simulink model "SIMULINK"  (R2023a)
settings: Solver=VariableStepAuto  StartTime=0.0  StopTime=STOP  MaxStep=0.1  MinStep=0.01  RelTol=1e-3
values from neighbouring files (symbols this model uses):
  a = pars(1,1)    [simulinkmodel.m]
  a1 = 0.02    [Izhikevich.m]    (also in simulinkmodel.m = pars(2,1))
  a2 = 0.1    [Izhikevich.m]    (also in simulinkmodel.m = pars(3,1))
  b = normalize(V_feedback)    [interconnection.m]    (also in simulinkmodel.m = pars(1,2))
  b1 = 0.2    [Izhikevich.m]    (also in simulinkmodel.m = pars(2,2))
  b2 = 0.2    [Izhikevich.m]    (also in simulinkmodel.m = pars(3,2))
  c = pars(1,3)    [simulinkmodel.m]
  c1 = -65    [Izhikevich.m]    (also in simulinkmodel.m = pars(2,3))
  c2 = -65    [Izhikevich.m]    (also in simulinkmodel.m = pars(3,3))
  d = pars(1,4)    [simulinkmodel.m]
  d1 = 8    [Izhikevich.m]    (also in simulinkmodel.m = pars(2,4))
  d2 = 2    [Izhikevich.m]    (also in simulinkmodel.m = pars(3,4))
  STOP = 500    [simulinkmodel.m]
settings Model: Creator=HP  LastModifiedBy=HP
settings SolverCC: InitialStep=Auto

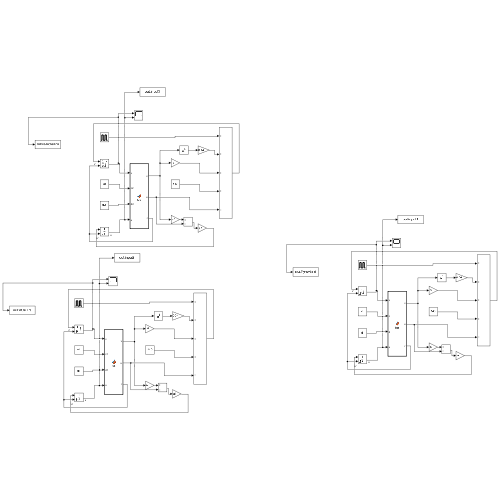
[thumbnail: Simulink's stored preview of the top-level diagram]
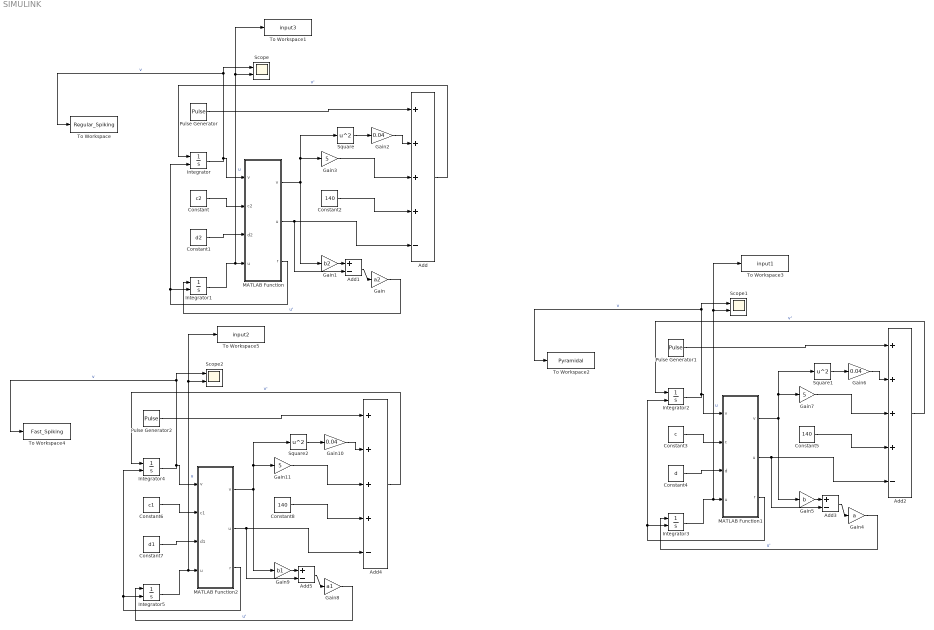
== system SIMULINK ==
  Add : Sum  Inputs=++++-
  Add1 : Sum  Inputs=+-
  Add2 : Sum  Inputs=++++-
  Add3 : Sum  Inputs=+-
  Add4 : Sum  Inputs=++++-
  Add5 : Sum  Inputs=+-
  Constant : Constant  Value=c2
  Constant1 : Constant  Value=d2
  Constant2 : Constant  Value=140
  Constant3 : Constant  Value=c
  Constant4 : Constant  Value=d
  Constant5 : Constant  Value=140
  Constant6 : Constant  Value=c1
  Constant7 : Constant  Value=d1
  Constant8 : Constant  Value=140
  Gain : Gain  Gain=a2
  Gain1 : Gain  Gain=b2
  Gain10 : Gain  Gain=0.04
  Gain11 : Gain  Gain=5
  Gain2 : Gain  Gain=0.04
  Gain3 : Gain  Gain=5
  Gain4 : Gain  Gain=a
  Gain5 : Gain  Gain=b
  Gain6 : Gain  Gain=0.04
  Gain7 : Gain  Gain=5
  Gain8 : Gain  Gain=a1
  Gain9 : Gain  Gain=b1
  Integrator : Integrator  ExternalReset=rising  InitialCondition=c  LimitOutput=on  UpperSaturationLimit=30
  Integrator1 : Integrator  ExternalReset=rising  InitialCondition=d
  Integrator2 : Integrator  ExternalReset=rising  InitialCondition=c  LimitOutput=on  UpperSaturationLimit=30
  Integrator3 : Integrator  ExternalReset=rising  InitialCondition=d
  Integrator4 : Integrator  ExternalReset=rising  InitialCondition=c  LimitOutput=on  UpperSaturationLimit=30
  Integrator5 : Integrator  ExternalReset=rising  InitialCondition=d
  MATLAB Function : MATLAB Function  TreatAsAtomicUnit=on
  MATLAB Function1 : MATLAB Function  TreatAsAtomicUnit=on
  MATLAB Function2 : MATLAB Function  TreatAsAtomicUnit=on
  Pulse Generator : DiscretePulseGenerator  PulseType=Time based  Amplitude=20  Period=STOP/2  PulseWidth=50  PhaseDelay=40
  Pulse Generator1 : DiscretePulseGenerator  PulseType=Time based  Amplitude=20  Period=STOP/2  PulseWidth=50  PhaseDelay=40
  Pulse Generator2 : DiscretePulseGenerator  PulseType=Time based  Amplitude=20  Period=STOP/2  PulseWidth=50  PhaseDelay=40
  Scope : Scope  NumInputPorts=2
  Scope1 : Scope  NumInputPorts=2
  Scope2 : Scope  NumInputPorts=2
  Square : Math  Operator=square
  Square1 : Math  Operator=square
  Square2 : Math  Operator=square
  To Workspace : ToWorkspace  VariableName=Regular_Spiking  SampleTime=-1
  To Workspace1 : ToWorkspace  VariableName=input3  SampleTime=-1
  To Workspace2 : ToWorkspace  VariableName=Pyramidal  SampleTime=-1
  To Workspace3 : ToWorkspace  VariableName=input1  SampleTime=-1
  To Workspace4 : ToWorkspace  VariableName=Fast_Spiking  SampleTime=-1
  To Workspace5 : ToWorkspace  VariableName=input2  SampleTime=-1
  wires:
  Integrator/1 -> To Workspace/1, Scope/1, MATLAB Function/1("v ")  "v"
  Add/1 -> Integrator/1  "v'"
  Gain/1 -> Integrator1/1  "u'"
  Square/1 -> Gain2/1
  Pulse Generator/1 -> Add/1
  Gain2/1 -> Add/2
  Gain3/1 -> Add/3
  Constant2/1 -> Add/4
  Gain1/1 -> Add1/1
  Add1/1 -> Gain/1
  Constant/1 -> MATLAB Function/2(c2)
  Constant1/1 -> MATLAB Function/3(d2)
  Integrator1/1 -> To Workspace1/1, Scope/2, MATLAB Function/4("u ")  "u"
  MATLAB Function/1(v) -> Gain1/1, Gain3/1, Square/1
  MATLAB Function/2(u) -> Add1/2, Add/5
  MATLAB Function/3(r) -> Integrator/2, Integrator1/2
  Integrator2/1 -> To Workspace2/1, Scope1/1, MATLAB Function1/1("v ")  "v"
  MATLAB Function1/3(r) -> Integrator2/2, Integrator3/2
  MATLAB Function1/2(u) -> Add3/2, Add2/5
  Constant5/1 -> Add2/4
  MATLAB Function1/1(v) -> Gain5/1, Gain7/1, Square1/1
  Gain5/1 -> Add3/1
  Add2/1 -> Integrator2/1  "v'"
  Gain6/1 -> Add2/2
  Add3/1 -> Gain4/1
  Square1/1 -> Gain6/1
  Constant4/1 -> MATLAB Function1/3(d)
  Constant3/1 -> MATLAB Function1/2(c)
  Integrator3/1 -> To Workspace3/1, Scope1/2, MATLAB Function1/4("u ")  "u"
  Pulse Generator1/1 -> Add2/1
  Gain4/1 -> Integrator3/1  "u'"
  Gain7/1 -> Add2/3
  Integrator4/1 -> To Workspace4/1, Scope2/1, MATLAB Function2/1("v ")  "v"
  MATLAB Function2/3(r) -> Integrator4/2, Integrator5/2
  MATLAB Function2/2(u) -> Add5/2, Add4/5
  Constant8/1 -> Add4/4
  MATLAB Function2/1(v) -> Gain9/1, Gain11/1, Square2/1
  Gain9/1 -> Add5/1
  Add4/1 -> Integrator4/1  "v'"
  Gain10/1 -> Add4/2
  Add5/1 -> Gain8/1
  Square2/1 -> Gain10/1
  Constant7/1 -> MATLAB Function2/3(d1)
  Constant6/1 -> MATLAB Function2/2(c1)
  Integrator5/1 -> To Workspace5/1, Scope2/2, MATLAB Function2/4("u ")  "u"
  Pulse Generator2/1 -> Add4/1
  Gain8/1 -> Integrator5/1  "u'"
  Gain11/1 -> Add4/3

== matlab function SIMULINK/MATLAB Function1 ==
  data: v input; c input; d input; u input; v output; u output; r output
function [v,u,r] = fcn(v,c,d,u)

if v >= 30
    v = c;
    u = c + d;
    r = 1;
else
    r = 0;
end

== matlab function SIMULINK/MATLAB Function ==
  data: v input; c2 input; d2 input; u input; v output; u output; r output
function [v,u,r] = fcn(v,c2,d2,u)

if v >= 30
    v = c2;
    u = c2 + d2;
    r = 1;
else
    r = 0;
end

== matlab function SIMULINK/MATLAB Function2 ==
  data: v input; c1 input; d1 input; u input; v output; u output; r output
function [v,u,r] = fcn(v,c1,d1,u)

if v >= 30
    v = c1;
    u = c1 + d1;
    r = 1;
else
    r = 0;
end
